simulink model "untitled"  (R2019b)
settings: Solver=VariableStepAuto  StartTime=0.0  StopTime=10.0  RelTol=1e-3
undefined symbols (not defined in the file): a1, a2, a3, b1, b2, b3, c1, c2, c3
settings Model: Creator=Inspiron  LastModifiedBy=Inspiron

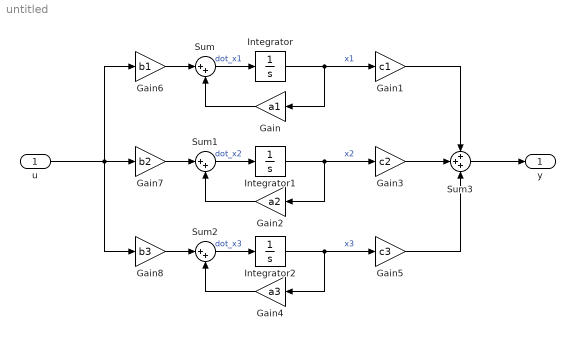
== system untitled ==
  u : Inport
  Gain : Gain  Gain=a1
  Gain1 : Gain  Gain=c1
  Gain2 : Gain  Gain=a2
  Gain3 : Gain  Gain=c2
  Gain4 : Gain  Gain=a3
  Gain5 : Gain  Gain=c3
  Gain6 : Gain  Gain=b1
  Gain7 : Gain  Gain=b2
  Gain8 : Gain  Gain=b3
  Integrator : Integrator
  Integrator1 : Integrator
  Integrator2 : Integrator
  Sum : Sum  Inputs=|++
  Sum1 : Sum  Inputs=|++
  Sum2 : Sum  Inputs=|++
  Sum3 : Sum  Inputs=+++
  y : Outport
  wires:
  Sum/1 -> Integrator/1  "dot_x1"
  Gain/1 -> Sum/2
  Integrator/1 -> Gain1/1, Gain/1  "x1"
  Gain2/1 -> Sum1/2
  Sum1/1 -> Integrator1/1  "dot_x2"
  Integrator1/1 -> Gain3/1, Gain2/1  "x2"
  Gain4/1 -> Sum2/2
  Sum2/1 -> Integrator2/1  "dot_x3"
  Integrator2/1 -> Gain5/1, Gain4/1  "x3"
  u/1 -> Gain6/1, Gain7/1, Gain8/1
  Gain1/1 -> Sum3/1
  Gain3/1 -> Sum3/2
  Gain5/1 -> Sum3/3
  Sum3/1 -> y/1
  Gain6/1 -> Sum/1
  Gain7/1 -> Sum1/1
  Gain8/1 -> Sum2/1
